simulink model "PID_outer"  (R2022a)
settings: Solver=VariableStepAuto  StartTime=0.0  StopTime=10  FixedStep=0.1  RelTol=1e-3
values from neighbouring files (symbols this model uses):
  den_c = C.den{:}    [outerloop_design_simulation.m]    (also in runscript_simulink.m)
  den_d = C_d.den{:}    [outerloop_design_simulation.m]    (also in runscript_simulink.m)
  freq_w = 2*pi*freq_hz    (= 1.0471975512)    [outerloop_design_simulation.m]    (also in runscript_simulink.m = 2.51327412287)
  num_c = C.num{:}    [outerloop_design_simulation.m]    (also in runscript_simulink.m)
  num_d = C_d.num{:}    [outerloop_design_simulation.m]    (also in runscript_simulink.m)
  radius = 0    [outerloop_design_simulation.m]    (also in runscript_simulink.m = 0.05)
  sat_lb = -(pi/180)*5    (= -0.0872664625997)    [outerloop_design_simulation.m]    (also in runscript_simulink.m)
  sat_ub = (pi/180)*5    (= 0.0872664625997)    [outerloop_design_simulation.m]    (also in runscript_simulink.m)
  sys_den = sys_tf1.den{:}    [outerloop_design_simulation.m]    (also in runscript_simulink.m)
  sys_num = sys_tf1.num{:}    [outerloop_design_simulation.m]    (also in runscript_simulink.m)
  Ts = 0.1    [PID_fromLQRscript.m]    (also in michiel_implementation.m; outerloop_design_simulation.m = 0.035; runscript_simulink.m = 0.01)
libraries: slpidlib x2
settings Model: Creator=michi  LastModifiedBy=michi

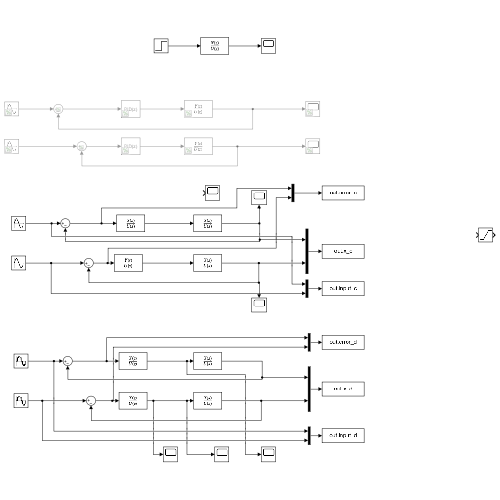
[thumbnail: Simulink's stored preview of the top-level diagram]
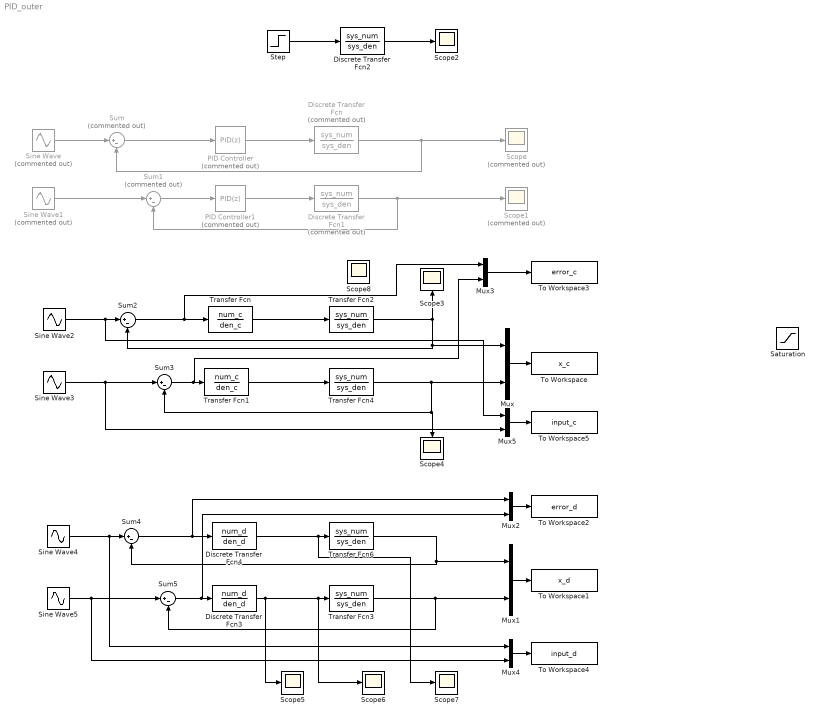
== system PID_outer ==
  Discrete Transfer Fcn : DiscreteTransferFcn  Commented=on  Numerator=sys_num  Denominator=sys_den
  Discrete Transfer Fcn1 : DiscreteTransferFcn  Commented=on  Numerator=sys_num  Denominator=sys_den
  Discrete Transfer Fcn2 : DiscreteTransferFcn  Numerator=sys_num  Denominator=sys_den
  Discrete Transfer Fcn3 : DiscreteTransferFcn  Numerator=num_d  Denominator=den_d  SampleTime=Ts
  Discrete Transfer Fcn4 : DiscreteTransferFcn  Numerator=num_d  Denominator=den_d  SampleTime=Ts
  Mux{,1..5} (6 alike) : Mux  Inputs=2
  PID Controller : slpidlib/PID Controller  Commented=on  Controller=PID  Form=Parallel  TimeDomain=Discrete-time  UseExternalTs=off  SampleTime=-1  IntegratorMethod=Forward Euler  FilterMethod=Forward Euler  ControllerParametersSource=internal  P=-1.936443475217614  I=-0.135033336384846  UseKiTs=off  D=-1.050533058102811  N=1/0.072016287542931  UseFilter=on  TunerSelectOption=Transfer Function Based (PID Tuner App)  InitialConditionSource=internal  InitialConditionForIntegrator=0  InitialConditionForFilter=0  DifferentiatorICPrevScaledInput=0  ExternalReset=none  TrackingMode=off  Kt=1  LimitOutput=off  SatLimitsSource=internal  UpperSaturationLimit=inf  LowerSaturationLimit=-inf  LinearizeAsGain=on  AntiWindupMode=none  Kb=1  POutMin=[]  POutMax=[]  IOutMin=[]  IOutMax=[]  DOutMin=[]  DOutMax=[]  NOutMin=[]  NOutMax=[]  SumOutMin=[]  SumOutMax=[]  SaturationOutMin=[]  SaturationOutMax=[]  PParamMin=[]  PParamMax=[]  IParamMin=[]  IParamMax=[]  DParamMin=[]  DParamMax=[]  NParamMin=[]  NParamMax=[]  KbParamMin=[]  KbParamMax=[]  KtParamMin=[]  KtParamMax=[]  KbOutMin=[]  KbOutMax=[]  KtOutMin=[]  KtOutMax=[]  IntegratorOutMin=[]  IntegratorOutMax=[]  FilterOutMin=[]  FilterOutMax=[]  SumI1OutMin=[]  SumI1OutMax=[]  SumI2OutMin=[]  SumI2OutMax=[]  SumI3OutMin=[]  SumI3OutMax=[]  SumI4OutMin=[]  SumI4OutMax=[]  SumDOutMin=[]  SumDOutMax=[]  DifferentiatorOutMin=[]  DifferentiatorOutMax=[]  FilterDiffOutCoefMin=[]  FilterDiffOutCoefMax=[]  ReciprocalOutMin=[]  ReciprocalOutMax=[]  SumDenOutMin=[]  SumDenOutMax=[]  SumNumOutMin=[]  SumNumOutMax=[]  DivideOutMin=[]  DivideOutMax=[]  UdiffTsProdOutMin=[]  UdiffTsProdOutMax=[]  NTsProdOutMin=[]  NTsProdOutMax=[]  UintegralTsProdOutMin=[]  UintegralTsProdOutMax=[]  UngainTsProdOutMin=[]  UngainTsProdOutMax=[]  IntegratorContinuousStateAttributes=''  IntegratorStateMustResolveToSignalObject=off  IntegratorRTWStateStorageClass=Auto  FilterContinuousStateAttributes=''  FilterStateMustResolveToSignalObject=off  FilterRTWStateStorageClass=Auto  ParallelPVariant=InternalParameters  IdealPVariant=Disabled  IVariant=InternalParameters  DVariant=InternalParameters  IntegratorVariant=Discrete  SatVariant=Disabled  AWVariant=Passthrough  PCopyVariant=Disabled  TRVariant=Disabled  FdbkBlocksVariant=Forward  IdealPFdbkVariant=Disabled  SatFdbkVariant=Disabled  DerivativeFilterVariant=ForwardEulerFilter  NVariant=InternalParameters  NCopyVariant=Disabled  FilterICVariant=InternalICsFilter  IntegratorICVariant=InternalICs  ExternalResetVariant=Disabled  TRSumVariant=Passthrough  SumFdbkVariant=Disabled  SumVariant=Sum_PID  TsampFilterVariant=InternalTs  TsampNgainVariant=Passthrough  TsampIntegralVariant=Passthrough  ExternalSaturationOutDataTypeStr=Inherit: Same as second input  aMode=0
  PID Controller1 : slpidlib/PID Controller  Commented=on  Controller=PID  Form=Parallel  TimeDomain=Discrete-time  UseExternalTs=off  SampleTime=-1  IntegratorMethod=Forward Euler  FilterMethod=Forward Euler  ControllerParametersSource=internal  P=-1.936443475217614  I=-0.135033336384846  UseKiTs=off  D=-1.050533058102811  N=1/0.072016287542931  UseFilter=on  TunerSelectOption=Transfer Function Based (PID Tuner App)  InitialConditionSource=internal  InitialConditionForIntegrator=0  InitialConditionForFilter=0  DifferentiatorICPrevScaledInput=0  ExternalReset=none  TrackingMode=off  Kt=1  LimitOutput=off  SatLimitsSource=internal  UpperSaturationLimit=inf  LowerSaturationLimit=-inf  LinearizeAsGain=on  AntiWindupMode=none  Kb=1  POutMin=[]  POutMax=[]  IOutMin=[]  IOutMax=[]  DOutMin=[]  DOutMax=[]  NOutMin=[]  NOutMax=[]  SumOutMin=[]  SumOutMax=[]  SaturationOutMin=[]  SaturationOutMax=[]  PParamMin=[]  PParamMax=[]  IParamMin=[]  IParamMax=[]  DParamMin=[]  DParamMax=[]  NParamMin=[]  NParamMax=[]  KbParamMin=[]  KbParamMax=[]  KtParamMin=[]  KtParamMax=[]  KbOutMin=[]  KbOutMax=[]  KtOutMin=[]  KtOutMax=[]  IntegratorOutMin=[]  IntegratorOutMax=[]  FilterOutMin=[]  FilterOutMax=[]  SumI1OutMin=[]  SumI1OutMax=[]  SumI2OutMin=[]  SumI2OutMax=[]  SumI3OutMin=[]  SumI3OutMax=[]  SumI4OutMin=[]  SumI4OutMax=[]  SumDOutMin=[]  SumDOutMax=[]  DifferentiatorOutMin=[]  DifferentiatorOutMax=[]  FilterDiffOutCoefMin=[]  FilterDiffOutCoefMax=[]  ReciprocalOutMin=[]  ReciprocalOutMax=[]  SumDenOutMin=[]  SumDenOutMax=[]  SumNumOutMin=[]  SumNumOutMax=[]  DivideOutMin=[]  DivideOutMax=[]  UdiffTsProdOutMin=[]  UdiffTsProdOutMax=[]  NTsProdOutMin=[]  NTsProdOutMax=[]  UintegralTsProdOutMin=[]  UintegralTsProdOutMax=[]  UngainTsProdOutMin=[]  UngainTsProdOutMax=[]  IntegratorContinuousStateAttributes=''  IntegratorStateMustResolveToSignalObject=off  IntegratorRTWStateStorageClass=Auto  FilterContinuousStateAttributes=''  FilterStateMustResolveToSignalObject=off  FilterRTWStateStorageClass=Auto  ParallelPVariant=InternalParameters  IdealPVariant=Disabled  IVariant=InternalParameters  DVariant=InternalParameters  IntegratorVariant=Discrete  SatVariant=Disabled  AWVariant=Passthrough  PCopyVariant=Disabled  TRVariant=Disabled  FdbkBlocksVariant=Forward  IdealPFdbkVariant=Disabled  SatFdbkVariant=Disabled  DerivativeFilterVariant=ForwardEulerFilter  NVariant=InternalParameters  NCopyVariant=Disabled  FilterICVariant=InternalICsFilter  IntegratorICVariant=InternalICs  ExternalResetVariant=Disabled  TRSumVariant=Passthrough  SumFdbkVariant=Disabled  SumVariant=Sum_PID  TsampFilterVariant=InternalTs  TsampNgainVariant=Passthrough  TsampIntegralVariant=Passthrough  ExternalSaturationOutDataTypeStr=Inherit: Same as second input  aMode=0
  Saturation : Saturate  UpperLimit=sat_ub  LowerLimit=sat_lb
  Scope : Scope  Commented=on
  Scope1 : Scope  Commented=on
  Scope{2..8} (7 alike) : Scope
  Sine Wave : Sin  Commented=on  Amplitude=0.1  Frequency=2*pi*0.25  Phase=pi/2  SampleTime=0
  Sine Wave1 : Sin  Commented=on  Amplitude=0.1  Frequency=2*pi*0.25  SampleTime=0
  Sine Wave2 : Sin  Amplitude=radius  Frequency=freq_w  Phase=pi/2  SampleTime=0
  Sine Wave3 : Sin  Amplitude=radius  Frequency=freq_w  SampleTime=0
  Sine Wave4 : Sin  Amplitude=radius  Frequency=freq_w  Phase=pi/2  SampleTime=Ts
  Sine Wave5 : Sin  Amplitude=radius  Frequency=freq_w  SampleTime=Ts
  Step : Step  SampleTime=0
  Sum : Sum  Commented=on  Inputs=|+-
  Sum1 : Sum  Commented=on  Inputs=|+-
  Sum{2..5} (4 alike) : Sum  Inputs=|+-
  To Workspace : ToWorkspace  VariableName=x_c  SampleTime=-1
  To Workspace1 : ToWorkspace  VariableName=x_d  SampleTime=-1
  To Workspace2 : ToWorkspace  VariableName=error_d  SampleTime=-1
  To Workspace3 : ToWorkspace  VariableName=error_c  SampleTime=-1
  To Workspace4 : ToWorkspace  VariableName=input_d  SampleTime=-1
  To Workspace5 : ToWorkspace  VariableName=input_c  SampleTime=-1
  Transfer Fcn : TransferFcn  Numerator=num_c  Denominator=den_c
  Transfer Fcn1 : TransferFcn  Numerator=num_c  Denominator=den_c
  Transfer Fcn{2..4,6} (4 alike) : TransferFcn  Numerator=sys_num  Denominator=sys_den
  wires:
  PID Controller/1 -> Discrete Transfer Fcn/1
  PID Controller1/1 -> Discrete Transfer Fcn1/1
  Sum1/1 -> PID Controller1/1
  Sum/1 -> PID Controller/1
  Discrete Transfer Fcn/1 -> Scope/1, Sum/2
  Discrete Transfer Fcn1/1 -> Scope1/1, Sum1/2
  Sine Wave/1 -> Sum/1
  Sine Wave1/1 -> Sum1/1
  Step/1 -> Discrete Transfer Fcn2/1
  Discrete Transfer Fcn2/1 -> Scope2/1
  Mux/1 -> To Workspace/1
  Mux1/1 -> To Workspace1/1
  Sine Wave4/1 -> Sum4/1, Mux4/1
  Sine Wave5/1 -> Sum5/1, Mux4/2
  Sum4/1 -> Mux2/1, Discrete Transfer Fcn4/1
  Transfer Fcn6/1 -> Sum4/2, Mux1/1
  Transfer Fcn3/1 -> Sum5/2, Mux1/2
  Sum5/1 -> Mux2/2, Discrete Transfer Fcn3/1
  Mux2/1 -> To Workspace2/1
  Discrete Transfer Fcn3/1 -> Scope6/1, Transfer Fcn3/1, Scope5/1
  Sum3/1 -> Mux3/2, Transfer Fcn1/1
  Mux3/1 -> To Workspace3/1
  Sum2/1 -> Mux3/1, Transfer Fcn/1
  Transfer Fcn2/1 -> Sum2/2, Mux/1, Scope3/1
  Transfer Fcn4/1 -> Sum3/2, Scope4/1, Mux/2
  Mux4/1 -> To Workspace4/1
  Discrete Transfer Fcn4/1 -> Scope7/1, Transfer Fcn6/1
  Transfer Fcn/1 -> Transfer Fcn2/1
  Transfer Fcn1/1 -> Transfer Fcn4/1
  Sine Wave3/1 -> Mux5/2, Sum3/1
  Mux5/1 -> To Workspace5/1
  Sine Wave2/1 -> Mux5/1, Sum2/1
